simulink model "Motor_Pos1"  (R2023b)
settings: Solver=ode45  StartTime=0.0  StopTime=10.0  RelTol=1e-3
settings Model: Creator=sansh  LastModifiedBy=barny
settings SolverCC: AlgebraicLoopSolver=TrustRegion
settings DataIOCC: ReturnWorkspaceOutputs=off
settings DebuggingCC: UnconnectedInputMsg=warning  UnconnectedOutputMsg=warning  UnconnectedLineMsg=warning  ArithmeticOperatorsInVariantConditions=warning
settings ModelReferenceCC: EnableRefExpFcnMdlSchedulingChecks=on
settings SFSimCC: SimUseLocalCustomCode=off  CustomCodeUndefinedFunction=UseInterfaceOnly
settings RTWCC: RTWUseLocalCustomCode=off
settings CodeAppCC: StateflowObjectComments=on

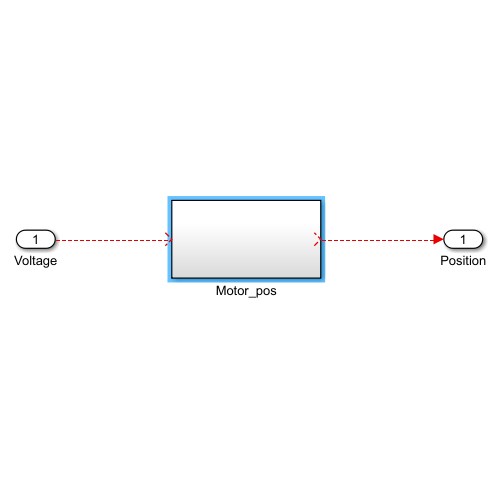
[thumbnail: Simulink's stored preview of the top-level diagram]
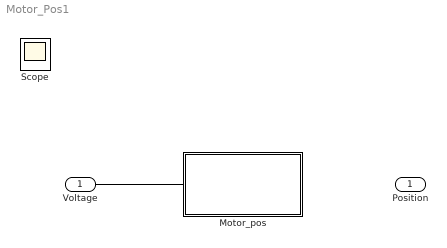
== system Motor_Pos1 ==
  Voltage : Inport
  Motor_pos : Subsystem
  Position : Outport
  Scope : Scope
  wires:
  Voltage/1 -> ?
  ? -> Position/1

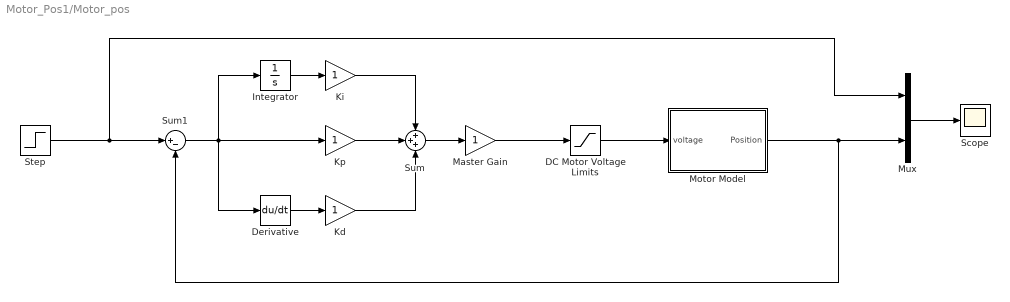
== system Motor_Pos1/Motor_pos ==
  DC Motor Voltage Limits : Saturate  UpperLimit=12  LowerLimit=-12
  Derivative : Derivative
  Integrator : Integrator
  Kd : Gain
  Ki : Gain
  Kp : Gain
  Master Gain : Gain
  Motor Model : Subsystem
  Mux : Mux  Inputs=2
  Scope : Scope
  Step : Step  SampleTime=0
  Sum : Sum  Inputs=+++
  Sum1 : Sum  Inputs=|+-
  wires:
  Motor Model/1(Position) -> Mux/2, Sum1/2
  Sum/1 -> Master Gain/1
  Sum1/1 -> Derivative/1, Integrator/1, Kp/1
  Kp/1 -> Sum/2
  Integrator/1 -> Ki/1
  Ki/1 -> Sum/1
  Step/1 -> Mux/1, Sum1/1
  Derivative/1 -> Kd/1
  Kd/1 -> Sum/3
  Mux/1 -> Scope/1
  Master Gain/1 -> DC Motor Voltage Limits/1
  DC Motor Voltage Limits/1 -> Motor Model/1(voltage)

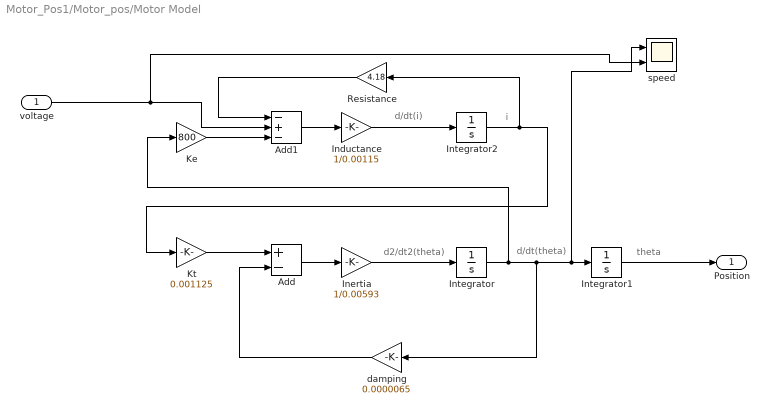
== system Motor_Pos1/Motor_pos/Motor Model ==
  note: i
  note: d/dt(i)
  note: d2/dt2(theta)
  note: d/dt(theta)
  note: theta
  voltage : Inport
  Add : Sum  Inputs=+-
  Add1 : Sum  Inputs=-+-
  Inductance : Gain  Gain=1/0.00115
  Inertia : Gain  Gain=1/0.00593
  Integrator : Integrator
  Integrator1 : Integrator
  Integrator2 : Integrator
  Ke : Gain  Gain=800
  Kt : Gain  Gain=0.001125
  Resistance : Gain  Gain=4.18
  damping : Gain  Gain=0.0000065
  speed : Scope  NumInputPorts=2
  Position : Outport
  wires:
  Integrator2/1 -> Resistance/1, Kt/1
  Inertia/1 -> Integrator/1
  damping/1 -> Add/2
  Integrator/1 -> Ke/1, damping/1, speed/1, Integrator1/1
  Ke/1 -> Add1/3
  Inductance/1 -> Integrator2/1
  Integrator1/1 -> Position/1
  Add/1 -> Inertia/1
  Resistance/1 -> Add1/1
  Add1/1 -> Inductance/1
  Kt/1 -> Add/1
  voltage/1 -> speed/2, Add1/2
